simulink model "NCMS_AltMis_항공대"  (R2022a)
settings: Solver=FixedStepAuto  StartTime=0.0  StopTime=inf  FixedStep=SampleTime  RelTol=1e-3
InitFcn:
  | NCMS_AltMis_Init;
values from neighbouring files (symbols this model uses):
  Kdpr = 0.004    [NCMS_AltMis_Init_항공대.m]
  Kdrr = 0.004    [NCMS_AltMis_Init_항공대.m]
  Kdvz = 0.0254    [NCMS_AltMis_Init_항공대.m]
  Kdyr = 0.0298    [NCMS_AltMis_Init_항공대.m]
  Kipr = 0.1    [NCMS_AltMis_Init_항공대.m]
  Kirr = 0.1    [NCMS_AltMis_Init_항공대.m]
  Kivx = 0.0728/g    (= 0.00742099898063)    [NCMS_AltMis_Init_항공대.m]
  Kivy = 0.0728/g    (= 0.00742099898063)    [NCMS_AltMis_Init_항공대.m]
  Kivz = 0.6304    [NCMS_AltMis_Init_항공대.m]
  Kix = 0.02    [NCMS_AltMis_Init_항공대.m]
  Kiyaxis = 0.02    [NCMS_AltMis_Init_항공대.m]
  Kiyr = 0.7395    [NCMS_AltMis_Init_항공대.m]
  Kiz = 0.09    [NCMS_AltMis_Init_항공대.m]
  Kpp = 3.3894    [NCMS_AltMis_Init_항공대.m]
  Kppr = 0.1    [NCMS_AltMis_Init_항공대.m]
  Kpr = 3.3894    [NCMS_AltMis_Init_항공대.m]
  Kprr = 0.1    [NCMS_AltMis_Init_항공대.m]
  Kpvx = 2.1109/g    (= 0.215178389399)    [NCMS_AltMis_Init_항공대.m]
  Kpvy = 2.1109/g    (= 0.215178389399)    [NCMS_AltMis_Init_항공대.m]
  Kpvz = 0.3191    [NCMS_AltMis_Init_항공대.m]
  Kpx = 1    [NCMS_AltMis_Init_항공대.m]
  Kpy = 3.3894    [NCMS_AltMis_Init_항공대.m]
  Kpyaxis = 1    [NCMS_AltMis_Init_항공대.m]
  Kpyr = 0.3744    [NCMS_AltMis_Init_항공대.m]
  Kpz = 2.4    [NCMS_AltMis_Init_항공대.m]
  LAND_PRES_VEL = 0.2    [NCMS_AltMis_Init_항공대.m]
  MAX_CONTROL_ANGLE_PITCH = 30*pi/180    (= 0.523598775598)    [Init_FLIGHT_Hexacopter.m]    (also in NCMS_AltMis_Init_항공대.m = 0.349065850399)
  MAX_CONTROL_ANGLE_RATE_PITCH = 360*pi/180    (= 6.28318530718)    [Init_FLIGHT_Hexacopter.m]    (also in NCMS_AltMis_Init_항공대.m)
  MAX_CONTROL_ANGLE_RATE_ROLL = 360*pi/180    (= 6.28318530718)    [Init_FLIGHT_Hexacopter.m]    (also in NCMS_AltMis_Init_항공대.m)
  MAX_CONTROL_ANGLE_RATE_Y = 120*pi/180    (= 2.09439510239)    [Init_FLIGHT_Hexacopter.m]    (also in NCMS_AltMis_Init_항공대.m)
  MAX_CONTROL_ANGLE_ROLL = 30*pi/180    (= 0.523598775598)    [Init_FLIGHT_Hexacopter.m]    (also in NCMS_AltMis_Init_항공대.m = 0.349065850399)
  MAX_CONTROL_VELOCITY_XY = 1.5    [Init_FLIGHT_Hexacopter.m]    (also in NCMS_AltMis_Init_항공대.m)
  MAX_CONTROL_VELOCITY_Z = 1    [Init_FLIGHT_Hexacopter.m]    (also in NCMS_AltMis_Init_항공대.m)
  Npr = 50    [NCMS_AltMis_Init_항공대.m]
  Nrr = 50    [NCMS_AltMis_Init_항공대.m]
  Nvz = Npr    (= 50)    [NCMS_AltMis_Init_항공대.m]
  Nyr = 50    [NCMS_AltMis_Init_항공대.m]
  SampleTime = 1/250    (= 0.004)    [Init_FLIGHT_Hexacopter.m]    (also in NCMS_AltMis_Init_항공대.m = 0.01)
  THR_HOVER = 0.6085    [NCMS_AltMis_Init_항공대.m]
  THR_IDLE = 0.2    [NCMS_AltMis_Init_항공대.m]
undefined symbols (not defined in the file or in its folder): dev, Kdz, Main, Nz, pwm_output0
libraries: slpidlib x15, simulink x9, px4Sensorslib x3, px4uORBlib x3, uavalgslib x2, px4lib x1
(part 3 of 3)

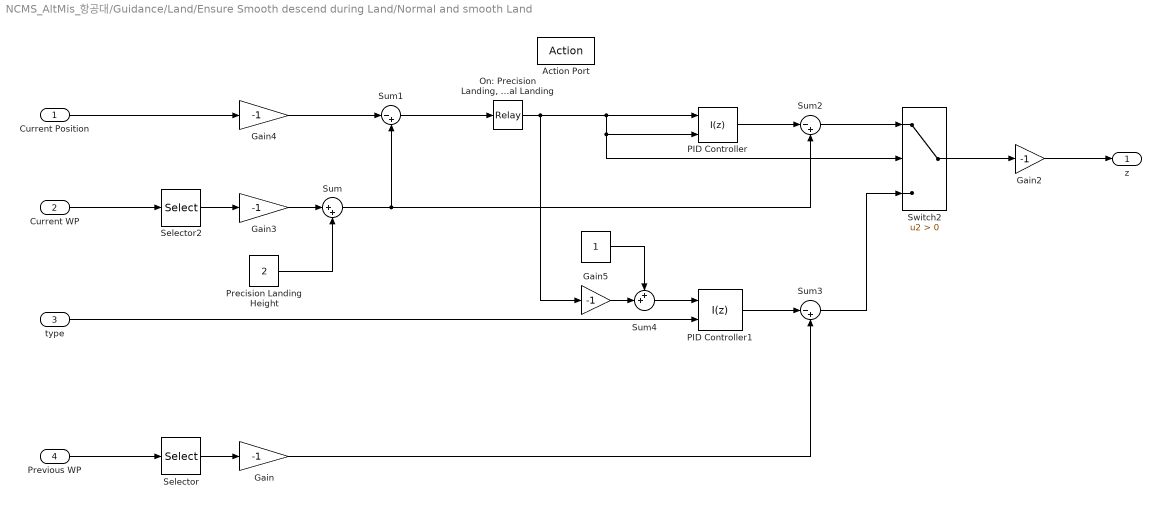
== system NCMS_AltMis_항공대/Guidance/Land/Ensure Smooth descend during Land/Normal and smooth Land ==
  Current Position : Inport
  Current WP : Inport  Port=2
  type : Inport  Port=3
  Previous WP : Inport  Port=4
  Action Port : ActionPort  ActionPortLabel=if(u1 > 0)
  " " : Constant  OutDataTypeStr=single
  Gain{,2..5} (5 alike) : Gain  Gain=-1
  "On: Precision Landing, Off: Normal Landing" : Relay  OnSwitchValue=0  OffSwitchValue=-1
  PID Controller : slpidlib/PID Controller  Controller=I  Form=Parallel  TimeDomain=Discrete-time  UseExternalTs=off  SampleTime=SampleTime  IntegratorMethod=Forward Euler  FilterMethod=Forward Euler  ControllerParametersSource=internal  P=1  I=LAND_PRES_VEL  UseKiTs=off  D=0  N=100  UseFilter=on  TunerSelectOption=Transfer Function Based (PID Tuner App)  InitialConditionSource=internal  InitialConditionForIntegrator=0  InitialConditionForFilter=0  DifferentiatorICPrevScaledInput=0  ExternalReset=either  TrackingMode=off  Kt=1  LimitOutput=on  SatLimitsSource=internal  UpperSaturationLimit=4  LowerSaturationLimit=0  LinearizeAsGain=on  AntiWindupMode=clamping  Kb=1  POutMin=[]  POutMax=[]  IOutMin=[]  IOutMax=[]  DOutMin=[]  DOutMax=[]  NOutMin=[]  NOutMax=[]  SumOutMin=[]  SumOutMax=[]  SaturationOutMin=[]  SaturationOutMax=[]  PParamMin=[]  PParamMax=[]  IParamMin=[]  IParamMax=[]  DParamMin=[]  DParamMax=[]  NParamMin=[]  NParamMax=[]  KbParamMin=[]  KbParamMax=[]  KtParamMin=[]  KtParamMax=[]  KbOutMin=[]  KbOutMax=[]  KtOutMin=[]  KtOutMax=[]  IntegratorOutMin=[]  IntegratorOutMax=[]  FilterOutMin=[]  FilterOutMax=[]  SumI1OutMin=[]  SumI1OutMax=[]  SumI2OutMin=[]  SumI2OutMax=[]  SumI3OutMin=[]  SumI3OutMax=[]  SumI4OutMin=[]  SumI4OutMax=[]  SumDOutMin=[]  SumDOutMax=[]  DifferentiatorOutMin=[]  DifferentiatorOutMax=[]  FilterDiffOutCoefMin=[]  FilterDiffOutCoefMax=[]  ReciprocalOutMin=[]  ReciprocalOutMax=[]  SumDenOutMin=[]  SumDenOutMax=[]  SumNumOutMin=[]  SumNumOutMax=[]  DivideOutMin=[]  DivideOutMax=[]  UdiffTsProdOutMin=[]  UdiffTsProdOutMax=[]  NTsProdOutMin=[]  NTsProdOutMax=[]  UintegralTsProdOutMin=[]  UintegralTsProdOutMax=[]  UngainTsProdOutMin=[]  UngainTsProdOutMax=[]  IntegratorContinuousStateAttributes=''  IntegratorStateMustResolveToSignalObject=off  IntegratorRTWStateStorageClass=Auto  FilterContinuousStateAttributes=''  FilterStateMustResolveToSignalObject=off  FilterRTWStateStorageClass=Auto  ParallelPVariant=Disabled  IdealPVariant=Disabled  IVariant=InternalParameters  DVariant=Disabled  IntegratorVariant=Discrete  SatVariant=Enabled  AWVariant=DiscClampingParallel  PCopyVariant=Disabled  TRVariant=Disabled  FdbkBlocksVariant=Forward  IdealPFdbkVariant=Disabled  SatFdbkVariant=Disabled  DerivativeFilterVariant=Disabled  NVariant=Disabled  NCopyVariant=Disabled_SignalSpec  FilterICVariant=Disabled  IntegratorICVariant=InternalICs  ExternalResetVariant=ExternalReset  TRSumVariant=Passthrough  SumFdbkVariant=Disabled  SumVariant=Passthrough_I  TsampFilterVariant=InternalTs  TsampNgainVariant=Passthrough  TsampIntegralVariant=Passthrough  ExternalSaturationOutDataTypeStr=Inherit: Same as second input  aMode=0
  PID Controller1 : slpidlib/PID Controller  Controller=I  Form=Parallel  TimeDomain=Discrete-time  UseExternalTs=off  SampleTime=SampleTime  IntegratorMethod=Forward Euler  FilterMethod=Forward Euler  ControllerParametersSource=internal  P=1  I=MAX_CONTROL_VELOCITY_Z  UseKiTs=off  D=0  N=100  UseFilter=on  TunerSelectOption=Transfer Function Based (PID Tuner App)  InitialConditionSource=internal  InitialConditionForIntegrator=0  InitialConditionForFilter=0  DifferentiatorICPrevScaledInput=0  ExternalReset=either  TrackingMode=off  Kt=1  LimitOutput=on  SatLimitsSource=internal  UpperSaturationLimit=inf  LowerSaturationLimit=0  LinearizeAsGain=on  AntiWindupMode=clamping  Kb=1  POutMin=[]  POutMax=[]  IOutMin=[]  IOutMax=[]  DOutMin=[]  DOutMax=[]  NOutMin=[]  NOutMax=[]  SumOutMin=[]  SumOutMax=[]  SaturationOutMin=[]  SaturationOutMax=[]  PParamMin=[]  PParamMax=[]  IParamMin=[]  IParamMax=[]  DParamMin=[]  DParamMax=[]  NParamMin=[]  NParamMax=[]  KbParamMin=[]  KbParamMax=[]  KtParamMin=[]  KtParamMax=[]  KbOutMin=[]  KbOutMax=[]  KtOutMin=[]  KtOutMax=[]  IntegratorOutMin=[]  IntegratorOutMax=[]  FilterOutMin=[]  FilterOutMax=[]  SumI1OutMin=[]  SumI1OutMax=[]  SumI2OutMin=[]  SumI2OutMax=[]  SumI3OutMin=[]  SumI3OutMax=[]  SumI4OutMin=[]  SumI4OutMax=[]  SumDOutMin=[]  SumDOutMax=[]  DifferentiatorOutMin=[]  DifferentiatorOutMax=[]  FilterDiffOutCoefMin=[]  FilterDiffOutCoefMax=[]  ReciprocalOutMin=[]  ReciprocalOutMax=[]  SumDenOutMin=[]  SumDenOutMax=[]  SumNumOutMin=[]  SumNumOutMax=[]  DivideOutMin=[]  DivideOutMax=[]  UdiffTsProdOutMin=[]  UdiffTsProdOutMax=[]  NTsProdOutMin=[]  NTsProdOutMax=[]  UintegralTsProdOutMin=[]  UintegralTsProdOutMax=[]  UngainTsProdOutMin=[]  UngainTsProdOutMax=[]  IntegratorContinuousStateAttributes=''  IntegratorStateMustResolveToSignalObject=off  IntegratorRTWStateStorageClass=Auto  FilterContinuousStateAttributes=''  FilterStateMustResolveToSignalObject=off  FilterRTWStateStorageClass=Auto  ParallelPVariant=Disabled  IdealPVariant=Disabled  IVariant=InternalParameters  DVariant=Disabled  IntegratorVariant=Discrete  SatVariant=Enabled  AWVariant=DiscClampingParallel  PCopyVariant=Disabled  TRVariant=Disabled  FdbkBlocksVariant=Forward  IdealPFdbkVariant=Disabled  SatFdbkVariant=Disabled  DerivativeFilterVariant=Disabled  NVariant=Disabled  NCopyVariant=Disabled_SignalSpec  FilterICVariant=Disabled  IntegratorICVariant=InternalICs  ExternalResetVariant=ExternalReset  TRSumVariant=Passthrough  SumFdbkVariant=Disabled  SumVariant=Passthrough_I  TsampFilterVariant=InternalTs  TsampNgainVariant=Passthrough  TsampIntegralVariant=Passthrough  ExternalSaturationOutDataTypeStr=Inherit: Same as second input  aMode=0
  Precision Landing Height : Constant  Value=2  OutDataTypeStr=single
  Selector : Selector  InputPortWidth=4  IndexOptions=Index vector (dialog)  Indices=[3]  OutputSizes=1
  Selector2 : Selector  InputPortWidth=4  IndexOptions=Index vector (dialog)  Indices=[3]  OutputSizes=1
  Sum : Sum  Inputs=|++
  Sum1 : Sum  Inputs=|-+
  Sum2 : Sum  Inputs=|-+
  Sum3 : Sum  Inputs=|-+
  Sum4 : Sum  Inputs=++|
  Switch2 : Switch  Criteria=u2 > Threshold  SaturateOnIntegerOverflow=off  InputSameDT=off
  z : Outport
  wires:
  "On: Precision Landing, Off: Normal Landing"/1 -> Gain5/1, PID Controller/1, PID Controller/2, Switch2/2
  Sum4/1 -> PID Controller1/1
  Selector/1 -> Gain/1
  Sum3/1 -> Switch2/3
  Sum/1 -> Sum2/2, Sum1/2
  Switch2/1 -> Gain2/1
  Sum1/1 -> "On: Precision Landing, Off: Normal Landing"/1
  PID Controller/1 -> Sum2/1
  Sum2/1 -> Switch2/1
  Selector2/1 -> Gain3/1
  Current Position/1 -> Gain4/1
  Gain5/1 -> Sum4/2
  Gain3/1 -> Sum/1
  Gain/1 -> Sum3/2
  Precision Landing Height/1 -> Sum/2
  " "/1 -> Sum4/1
  Gain2/1 -> z/1
  type/1 -> PID Controller1/2
  Previous WP/1 -> Selector/1
  Current WP/1 -> Selector2/1
  PID Controller1/1 -> Sum3/1
  Gain4/1 -> Sum1/1

== system NCMS_AltMis_항공대/Guidance/Land/Ensure Smooth descend during Land/Subsystem1 ==
  Current Position : Inport
  Current WP : Inport  Port=2
  Gain1 : Gain  Gain=-1
  Relay : Relay  OnSwitchValue=-2  OffSwitchValue=-4
  Selector4 : Selector  InputPortWidth=4  IndexOptions=Index vector (dialog)  Indices=[1 2]  OutputSizes=1
  Square Root : Sqrt
  Square1 : Math  Operator=square
  Subtract : Sum  Inputs=+-
  Sum of Elements : Sum  Inputs=+
  LAND RAD : Outport
  wires:
  Selector4/1 -> Subtract/2
  Current WP/1 -> Selector4/1
  Current Position/1 -> Subtract/1
  Relay/1 -> LAND RAD/1
  Subtract/1 -> Square1/1
  Sum of Elements/1 -> Square Root/1
  Square1/1 -> Sum of Elements/1
  Square Root/1 -> Gain1/1
  Gain1/1 -> Relay/1

== system NCMS_AltMis_항공대/Guidance/Land/Maintain Current Yaw during Land/Enabled Subsystem2 ==
  yaw_In : Inport
  Enable : EnablePort
  yaw_Out : Outport
  wires:
  yaw_In/1 -> yaw_Out/1

== system NCMS_AltMis_항공대/Guidance/Take-off/Maintain Current Yaw during TakeOff/Enabled Subsystem2 ==
  yaw_In : Inport
  Enable : EnablePort
  yaw_Out : Outport
  wires:
  yaw_In/1 -> yaw_Out/1

== matlab function NCMS_AltMis_항공대/Mixer/If Action Subsystem1/pwm_out2 ==
  data: Roll input; M1 output; Pitch input; Yaw input; Thrust input; M2 output; M3 output; M4 output
function [M1, M2, M3, M4] = motor_mixer(Roll, Pitch, Yaw, Thrust)
%Function description:
%  Control allocation. The quadrotor type is X-configuration,
%  and the airframe is as follows:
%3↓   1↑
 %  \ /
 %  / \
 %2↑   4↓
%Input：
%  Roll, Pitch, Yaw: attitude controller output.
%  Thrust

idle_PWM = 1000;
scale = 1000;

scale_att = scale*Thrust;

M1 = uint16(Thrust*scale + (- Roll + Pitch + Yaw) * scale_att + idle_PWM);
M2 = uint16(Thrust*scale + (Roll - Pitch + Yaw) * scale_att + idle_PWM);
M3 = uint16(Thrust*scale + (Roll + Pitch - Yaw) * scale_att + idle_PWM);
M4 = uint16(Thrust*scale + (- Roll - Pitch - Yaw) * scale_att + idle_PWM);

== matlab function NCMS_AltMis_항공대/Mixer/If Action Subsystem2/pwm_out2 ==
  data: Roll input; M1 output; Pitch input; Yaw input; Thrust input; M2 output; M3 output; M4 output
function [M1, M2, M3, M4] = motor_mixer(Roll, Pitch, Yaw, Thrust)
%Function description:
%  Control allocation. The quadrotor type is X-configuration,
%  and the airframe is as follows:
%3↓   1↑
 %  \ /
 %  / \
 %2↑   4↓
%Input：
%  Roll, Pitch, Yaw: attitude controller output.
%  Thrust

idle_PWM = 1000;
scale = 1000;

scale_att = scale;

M1 = uint16(Thrust*scale + (- Roll + Pitch + Yaw) * scale_att + idle_PWM);
M2 = uint16(Thrust*scale + (Roll - Pitch + Yaw) * scale_att + idle_PWM);
M3 = uint16(Thrust*scale + (Roll + Pitch - Yaw) * scale_att + idle_PWM);
M4 = uint16(Thrust*scale + (- Roll - Pitch - Yaw) * scale_att + idle_PWM);

== matlab function NCMS_AltMis_항공대/quat2eul ==
  data: q input; ypr output
function ypr  = quat2eul(q)

% Quaternion conversion to Euler angles based on the PX4 Firmware v1.10.2
% release.

phi = atan2(2*(q(1)*q(2) + q(3)* q(4)), q(1)^2 - q(2)^2 - q(3)^2 + q(4)^2);
theta = asin(-2*(q(2)*q(4) - q(1)*q(3)));
psi = atan2(2*(q(2)*q(3) + q(1)* q(4)), q(1)^2 + q(2)^2 - q(3)^2 - q(4)^2);

ypr = [psi theta phi];

end

== matlab function NCMS_AltMis_항공대/Read wapoints from Mission in QGC/Convert LLA to NED ==
  data: previous output; previousSetpoint input; currentSetpoint input; nextSetpoint input; homePosition input; current output; next output; type output
function [previous, current, next, type] = fcn(previousSetpoint, currentSetpoint, nextSetpoint, homePosition)
% previousSetpoint(1:5) = [previousSetpoint.lat, previousSetpoint.lon, previousSetpoint.alt, previousSetpoint.yaw, previousSetpoint.valid]
% currentSetpoint(1:6) = [currentSetpoint.lat, currentSetpoint.lon, currentSetpoint.alt, currentSetpoint.yaw, currentSetpoint.type, currentSetpoint.valid]
% nextSetpoint(1:5) = [nextSetpoint.lat, nextSetpoint.lon, nextSetpoint.alt, nextSetpoint.yaw, nextSetpoint.valid]
% homePosition(1:4) = [homePosition.lat, homePosition.lon, homePosition.alt, homePosition.valid_hpos]

previous = zeros(1,4);
current = zeros(1,4);
next = zeros(1,4);

lla0 = [homePosition(1), homePosition(2), homePosition(3)];
 
currentValid = homePosition(4) && currentSetpoint(6) && (currentSetpoint(5) ~= 5); % Avoid NED conversion when mission is not started yet and we receive IDLE setpoint
previousvalid = homePosition(4) && previousSetpoint(6);
nextValid = homePosition(4) && nextSetpoint(6);

type = [uint8(previousSetpoint(5)) uint8(currentSetpoint(5)) uint8(nextSetpoint(5))];

if(currentValid)
    lla = [currentSetpoint(1), currentSetpoint(2), currentSetpoint(3)];
    current = [lla2ned(lla,lla0,'flat'), currentSetpoint(4)];
end

if(previousvalid)
    lla = [previousSetpoint(1), previousSetpoint(2), previousSetpoint(3)];
    previous = [lla2ned(lla,lla0,'flat'), previousSetpoint(4)];
end

if(nextValid)
    lla = [nextSetpoint(1), nextSetpoint(2), nextSetpoint(3)];
    next = [lla2ned(lla,lla0,'flat'), nextSetpoint(4)];
end

== matlab function NCMS_AltMis_항공대/Postion Controller/Position Controller/MATLAB Function ==
  data: eaxy input; psi input; phi output; theta output
function [phi, theta] = fcn(eaxy, psi)
%Function description:
%  Convert the desired horizontal acceleration to the desired attitude angle
%Input:
%  eax, eaxy: desired horizontal acceleration
%  psi: yaw
%Output:
%  phi, theta: desired roll angle and desired pitch angle
eax = eaxy(1);
eay = eaxy(2);

phi = (-sin(psi)*eax + cos(psi)*eay);
theta = (-cos(psi)*eax - sin(psi)*eay);

== matlab function NCMS_AltMis_항공대/Mixer/If Action Subsystem/pwm_out2 ==
  data: Roll input; M1 output; Pitch input; Yaw input; Thrust input; M2 output; M3 output; M4 output
function [M1, M2, M3, M4] = motor_mixer(Roll, Pitch, Yaw, Thrust)
%Function description:
%  Control allocation. The quadrotor type is X-configuration,
%  and the airframe is as follows:
%3↓   1↑
 %  \ /
 %  / \
 %2↑   4↓
%Input：
%  Roll, Pitch, Yaw: attitude controller output.
%  Thrust

idle_PWM = 1000;
scale = 1000;

scale_att = scale*Thrust;

M1 = uint16(Thrust*scale + (- Roll + Pitch + Yaw) * scale_att + idle_PWM);
M2 = uint16(Thrust*scale + (Roll - Pitch + Yaw) * scale_att + idle_PWM);
M3 = uint16(Thrust*scale + (Roll + Pitch - Yaw) * scale_att + idle_PWM);
M4 = uint16(Thrust*scale + (- Roll - Pitch - Yaw) * scale_att + idle_PWM);
